simulink library "CTRL_LO_FRDIST"  (R2023b)
settings: Solver=VariableStepAuto  StartTime=0.0  StopTime=10.0  RelTol=1e-3
settings Model: Creator=blatak  LastModifiedBy=blatak

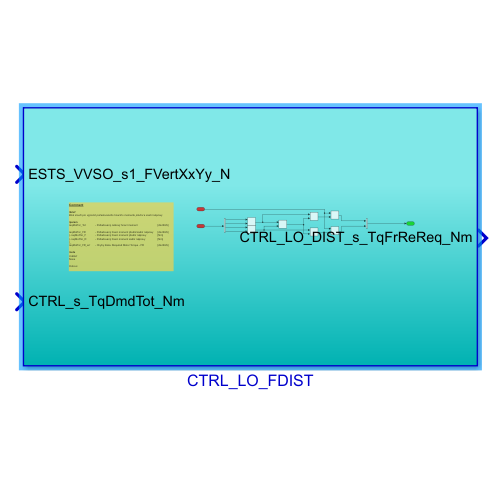
[thumbnail: Simulink's stored preview of the top-level diagram]
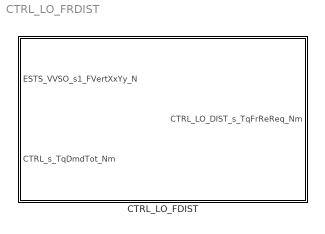
== system CTRL_LO_FRDIST ==
  CTRL_LO_FDIST : Subsystem

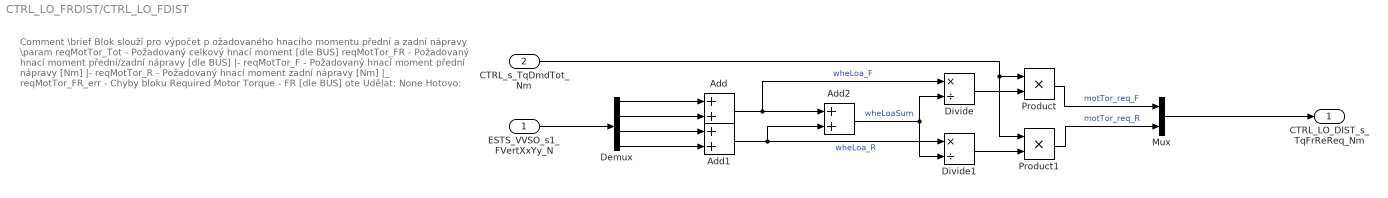
== system CTRL_LO_FRDIST/CTRL_LO_FDIST ==
  note: Comment
      |
      | \brief
      | Blok slouží pro výpočet p ožadovaného hnacího momentu přední a zadní nápravy
      |
      | \param
      | reqMotTor_Tot - Požadovaný celkový hnací moment [dle BUS]
      |
      | reqMotTor_FR - Požadovaný hnací moment přední/zadní nápravy [dle BUS]
      | |- reqMotTor_F - Požadovaný hnací moment přední nápravy [Nm]
      | |- reqMotTor_R - Požadovaný hnací moment zadní nápravy [Nm]
      | |_
      | reqMotTor_FR_err - Chyby bloku Required Motor Torque - FR [dle BUS]
      |
      | \note
      | Udělat:
      | None
      |
      | Hotovo:
  ESTS_VVSO_s1_FVertXxYy_N : Inport
  CTRL_s_TqDmdTot_Nm : Inport  Port=2
  Add : Sum
  Add1 : Sum
  Add2 : Sum
  Demux : Demux
  Divide : Product  Inputs=*/
  Divide1 : Product  Inputs=*/
  Mux : Mux  Inputs=2
  Product : Product
  Product1 : Product
  CTRL_LO_DIST_s_TqFrReReq_Nm : Outport
  wires:
  CTRL_s_TqDmdTot_Nm/1 -> Product1/1, Product/1
  ESTS_VVSO_s1_FVertXxYy_N/1 -> Demux/1
  Add/1 -> Divide/1, Add2/1  "wheLoa_F"
  Mux/1 -> CTRL_LO_DIST_s_TqFrReReq_Nm/1
  Add2/1 -> Divide/2, Divide1/2  "wheLoaSum"
  Divide1/1 -> Product1/2
  Product/1 -> Mux/1  "motTor_req_F"
  Add1/1 -> Add2/2, Divide1/1  "wheLoa_R"
  Product1/1 -> Mux/2  "motTor_req_R"
  Divide/1 -> Product/2
  Demux/1 -> Add/1
  Demux/4 -> Add1/2
  Demux/3 -> Add1/1
  Demux/2 -> Add/2
